simulink model "Decimator"  (R2023b)
settings: Solver=VariableStepAuto  StartTime=0.0  StopTime=10.0  RelTol=1e-3
PreLoadFcn:
  | startup
undefined symbols (not defined in the file): designMultirateFIR, fclk
libraries: hdlBasic x94, dspmlti4 x49, hdlsllib x2, simulink x2, dspbuff3 x2, dspsigops x2, hdlDSPIP x1, vmcUtilities x1
settings Model: Creator=andre  LastModifiedBy=andre

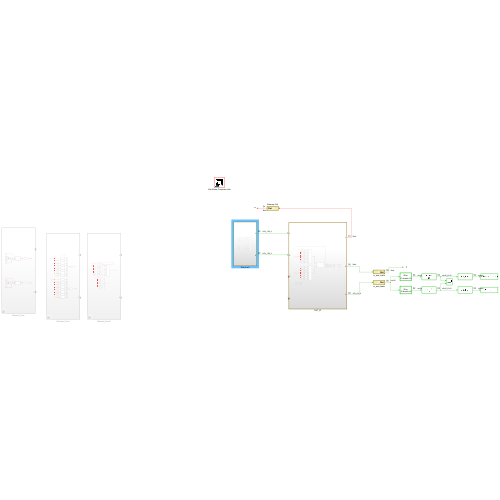
[thumbnail: Simulink's stored preview of the top-level diagram]
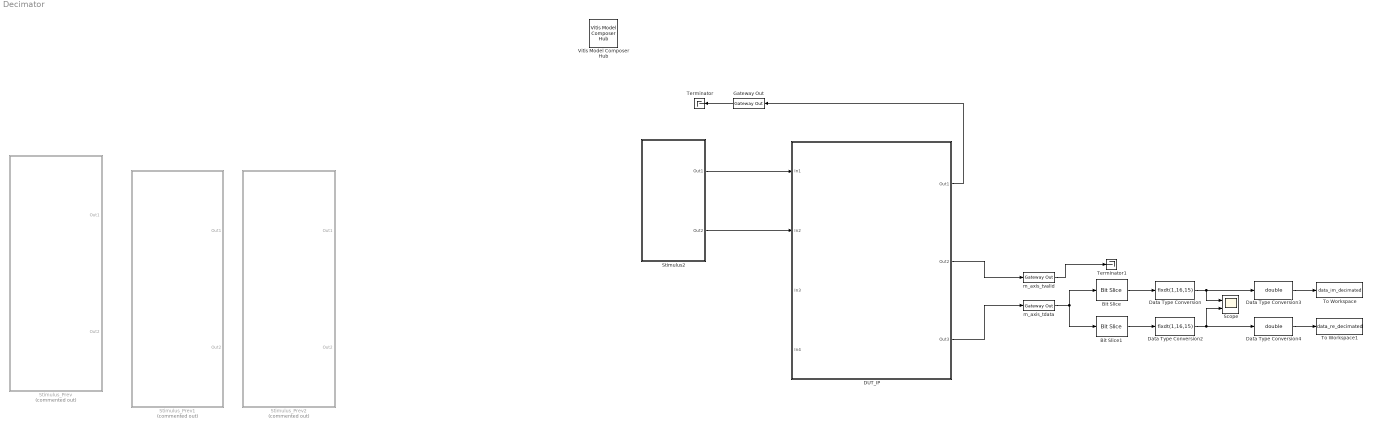
== system Decimator ==
  Bit Slice : hdlsllib/Logic and Bit Operations/Bit Slice  lidx=31  ridx=16
  Bit Slice1 : hdlsllib/Logic and Bit Operations/Bit Slice  lidx=15  ridx=0
  DUT_IP : Subsystem
  Data Type Conversion : DataTypeConversion  OutDataTypeStr=fixdt(1,16,15)  ConvertRealWorld=Stored Integer (SI)  SaturateOnIntegerOverflow=off  RndMeth=Floor
  Data Type Conversion2 : DataTypeConversion  OutDataTypeStr=fixdt(1,16,15)  ConvertRealWorld=Stored Integer (SI)  SaturateOnIntegerOverflow=off  RndMeth=Floor
  Data Type Conversion3 : DataTypeConversion  OutDataTypeStr=double  RndMeth=Floor
  Data Type Conversion4 : DataTypeConversion  OutDataTypeStr=double  RndMeth=Floor
  Gateway Out : hdlBasic/Gateway Out  inherit_from_input=off  hdl_port=on  rows=1  columns=1  UseAsDAC=off  DACChannel='1'  interface=None  automatic_assignment=on  address_offset=hex2dec('00')  intf_name=''  intf_description=''  timing_constraint=None  locs_specified=off  LOCs={}  io_standard={}  XmcBlockStatus=1  maskContainerNames=group4  block_type=gatewayout  block_config=sysgen:gateway_out_config  block_width_w=590  block_height_w=620  block_width=620  block_height=750
  Scope : Scope  NumInputPorts=2
  Stimulus2 : Subsystem
  Stimulus_Prev : Subsystem  Commented=on
  Stimulus_Prev1 : Subsystem  Commented=on
  Stimulus_Prev2 : Subsystem  Commented=on
  Terminator : Terminator
  Terminator1 : Terminator
  To Workspace : ToWorkspace  VariableName=data_im_decimated  SaveFormat=Timeseries  SampleTime=-1
  To Workspace1 : ToWorkspace  VariableName=data_re_decimated  SaveFormat=Timeseries  SampleTime=-1
  Vitis Model Composer Hub : vmcUtilities/Vitis Model Composer Hub  Tag=genX  CodeGeneration=off  SubsystemName=DUT_IP  DUTSubsystemName=DUT_IP  CompilationType=HDLCompilation  ExportTypeV2=IP Catalog  TargetDirectory=./netlist\ip\DUT_IP\src  exportDesign=on  analyzeDesign=off  validateDesignOnHw=off  ExportType=HDL  IpVendor=xilinx.com  IpLibrary=hls  IpVersion=1.0  IpHWLanguage=Verilog  AieCompilerOptions={}  AieSimulatorOptions={}  CreateTestbench=off  TestbenchStackSize=10  RunRtlSim=off  RunCSim=off  RunAieSim=off  AieSimTimeout=50000  RunAieSimProfiling=off  LaunchVitisAnalyzer=off  PlotOutput=off  RunX86Sim=off  X86SimTimeout=10  GenHwImage=off  GenLibadfXo=on  GenHwValidationCode=off  PlatformType=Not Specified  HwSystemType=Baremetal  HwValidationTarget=hw  ProjDevice=xczu28dr-ffvg1517-2-e  ProjDevicePart=xczu28dr-ffvg1517-2-e  SamplePeriod=-1  ClockFrequency=200  DataPathParallelism=1  xilinxfamily=zynquplusRFSOC  part=xczu28dr  speed=-2-e  package=ffvg1517  directory=./netlist\ip\DUT_IP\src  testbench=off  incr_netlist=off  synthesis_tool=Vivado  clock_wrapper=Clock Enables  dbl_ovrd=According to Block Masks  dcm_input_clock_period=10  sysclk_period=(1/fclk*8)*(1e6)  simulink_period=1/(fclk*8)  eval_field=0  IPInfoJsonString="{\"HDLSubsystem\":{\"SubsystemName\":\"DUT_IP\",\"IPName\":\"DUT_IP\",\"IPLibrary\":\"VMC\",\"IPVendor\":\"User Company\",\"IPVersion\":\"1.0\",\"TargetDirectory\":\"./netlist\",\"SubsystemDir\":\"./netlist\\\\ip\\\\DUT_IP\"},\"SubsystemTag\":\"HDLNode\"}"  LogFileName=''  NThreads=4
  m_axis_tdata : hdlBasic/Gateway Out  inherit_from_input=on  hdl_port=on  rows=1  columns=1  UseAsDAC=off  DACChannel='1'  interface=None  automatic_assignment=on  address_offset=hex2dec('00')  intf_name=''  intf_description=''  timing_constraint=None  locs_specified=off  LOCs={}  io_standard={}  XmcBlockStatus=1  maskContainerNames=group4  block_type=gatewayout  block_config=sysgen:gateway_out_config  block_width_w=590  block_height_w=620  block_width=620  block_height=750
  m_axis_tvalid : hdlBasic/Gateway Out  inherit_from_input=off  hdl_port=on  rows=1  columns=1  UseAsDAC=off  DACChannel='1'  interface=None  automatic_assignment=on  address_offset=hex2dec('00')  intf_name=''  intf_description=''  timing_constraint=None  locs_specified=off  LOCs={}  io_standard={}  XmcBlockStatus=1  maskContainerNames=group4  block_type=gatewayout  block_config=sysgen:gateway_out_config  block_width_w=590  block_height_w=620  block_width=620  block_height=750
  wires:
  Gateway Out/1 -> Terminator/1
  m_axis_tvalid/1 -> Terminator1/1
  m_axis_tdata/1 -> Bit Slice/1, Bit Slice1/1
  Bit Slice/1 -> Data Type Conversion/1
  Bit Slice1/1 -> Data Type Conversion2/1
  Data Type Conversion/1 -> Scope/1, Data Type Conversion3/1
  Data Type Conversion2/1 -> Scope/2, Data Type Conversion4/1
  Data Type Conversion3/1 -> To Workspace/1
  Data Type Conversion4/1 -> To Workspace1/1
  DUT_IP/1(Out1) -> Gateway Out/1
  DUT_IP/2(Out2) -> m_axis_tvalid/1
  DUT_IP/3(Out3) -> m_axis_tdata/1
  Stimulus2/1(Out1) -> DUT_IP/1(In1)
  Stimulus2/2(Out2) -> DUT_IP/2(In2)

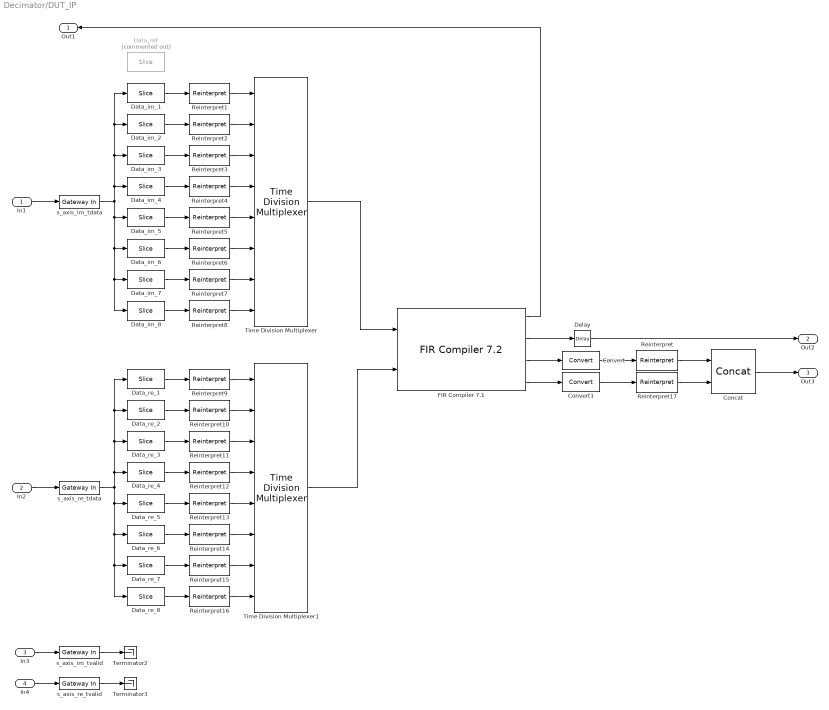
== system Decimator/DUT_IP ==
  In1 : Inport
  In2 : Inport  Port=2
  In3 : Inport  Port=3
  In4 : Inport  Port=4
  Concat : hdlBasic/Concat  num_inputs=2  XmcBlockStatus=1  maskContainerNames=group1  block_type=concat  block_config=sysgen:Concat_config
  Convert : hdlBasic/Convert  gui_display_data_type=Fixed-point  arith_type=Signed (2's comp)  n_bits=16  bin_pt=15  float_type=Single  exp_bits=8  fraction_bits=24  quantization=Truncate  overflow=Saturate  en=off  latency=1  pipeline=off  XmcBlockStatus=1  maskContainerNames=group2  block_type=convert  block_config=sysgen:Convert_config  block_width=595  block_height=885
  Convert1 : hdlBasic/Convert  gui_display_data_type=Fixed-point  arith_type=Signed (2's comp)  n_bits=16  bin_pt=15  float_type=Single  exp_bits=8  fraction_bits=24  quantization=Truncate  overflow=Saturate  en=off  latency=1  pipeline=off  XmcBlockStatus=1  maskContainerNames=group2  block_type=convert  block_config=sysgen:Convert_config  block_width=595  block_height=885
  Data_im_1 : hdlBasic/Slice  nbits=16  boolean_output=off  mode=Upper Bit Location + Width  bit1=127  base1=LSB of Input  bit0=16*8-(16*1)  base0=LSB of Input  XmcBlockStatus=1  maskContainerNames=group1  block_type=slice  block_config=sysgen:Slice_config
  Data_im_2 : hdlBasic/Slice  nbits=16  boolean_output=off  mode=Upper Bit Location + Width  bit1=111  base1=LSB of Input  bit0=16*8-(16*1)  base0=LSB of Input  XmcBlockStatus=1  maskContainerNames=group1  block_type=slice  block_config=sysgen:Slice_config
  Data_im_3 : hdlBasic/Slice  nbits=16  boolean_output=off  mode=Upper Bit Location + Width  bit1=95  base1=LSB of Input  bit0=16*8-(16*1)  base0=LSB of Input  XmcBlockStatus=1  maskContainerNames=group1  block_type=slice  block_config=sysgen:Slice_config
  Data_im_4 : hdlBasic/Slice  nbits=16  boolean_output=off  mode=Upper Bit Location + Width  bit1=79  base1=LSB of Input  bit0=16*8-(16*1)  base0=LSB of Input  XmcBlockStatus=1  maskContainerNames=group1  block_type=slice  block_config=sysgen:Slice_config
  Data_im_5 : hdlBasic/Slice  nbits=16  boolean_output=off  mode=Upper Bit Location + Width  bit1=63  base1=LSB of Input  bit0=16*8-(16*1)  base0=LSB of Input  XmcBlockStatus=1  maskContainerNames=group1  block_type=slice  block_config=sysgen:Slice_config
  Data_im_6 : hdlBasic/Slice  nbits=16  boolean_output=off  mode=Upper Bit Location + Width  bit1=47  base1=LSB of Input  bit0=16*8-(16*1)  base0=LSB of Input  XmcBlockStatus=1  maskContainerNames=group1  block_type=slice  block_config=sysgen:Slice_config
  Data_im_7 : hdlBasic/Slice  nbits=16  boolean_output=off  mode=Upper Bit Location + Width  bit1=31  base1=LSB of Input  bit0=16*8-(16*1)  base0=LSB of Input  XmcBlockStatus=1  maskContainerNames=group1  block_type=slice  block_config=sysgen:Slice_config
  Data_im_8 : hdlBasic/Slice  nbits=16  boolean_output=off  mode=Upper Bit Location + Width  bit1=15  base1=LSB of Input  bit0=16*8-(16*1)  base0=LSB of Input  XmcBlockStatus=1  maskContainerNames=group1  block_type=slice  block_config=sysgen:Slice_config
  Data_re_1 : hdlBasic/Slice  nbits=16  boolean_output=off  mode=Upper Bit Location + Width  bit1=127  base1=LSB of Input  bit0=16*8-(16*1)  base0=LSB of Input  XmcBlockStatus=1  maskContainerNames=group1  block_type=slice  block_config=sysgen:Slice_config
  Data_re_2 : hdlBasic/Slice  nbits=16  boolean_output=off  mode=Upper Bit Location + Width  bit1=111  base1=LSB of Input  bit0=16*8-(16*1)  base0=LSB of Input  XmcBlockStatus=1  maskContainerNames=group1  block_type=slice  block_config=sysgen:Slice_config
  Data_re_3 : hdlBasic/Slice  nbits=16  boolean_output=off  mode=Upper Bit Location + Width  bit1=95  base1=LSB of Input  bit0=16*8-(16*1)  base0=LSB of Input  XmcBlockStatus=1  maskContainerNames=group1  block_type=slice  block_config=sysgen:Slice_config
  Data_re_4 : hdlBasic/Slice  nbits=16  boolean_output=off  mode=Upper Bit Location + Width  bit1=79  base1=LSB of Input  bit0=16*8-(16*1)  base0=LSB of Input  XmcBlockStatus=1  maskContainerNames=group1  block_type=slice  block_config=sysgen:Slice_config
  Data_re_5 : hdlBasic/Slice  nbits=16  boolean_output=off  mode=Upper Bit Location + Width  bit1=63  base1=LSB of Input  bit0=16*8-(16*1)  base0=LSB of Input  XmcBlockStatus=1  maskContainerNames=group1  block_type=slice  block_config=sysgen:Slice_config
  Data_re_6 : hdlBasic/Slice  nbits=16  boolean_output=off  mode=Upper Bit Location + Width  bit1=47  base1=LSB of Input  bit0=16*8-(16*1)  base0=LSB of Input  XmcBlockStatus=1  maskContainerNames=group1  block_type=slice  block_config=sysgen:Slice_config
  Data_re_7 : hdlBasic/Slice  nbits=16  boolean_output=off  mode=Upper Bit Location + Width  bit1=31  base1=LSB of Input  bit0=16*8-(16*1)  base0=LSB of Input  XmcBlockStatus=1  maskContainerNames=group1  block_type=slice  block_config=sysgen:Slice_config
  Data_re_8 : hdlBasic/Slice  nbits=16  boolean_output=off  mode=Upper Bit Location + Width  bit1=15  base1=LSB of Input  bit0=16*8-(16*1)  base0=LSB of Input  XmcBlockStatus=1  maskContainerNames=group1  block_type=slice  block_config=sysgen:Slice_config
  Data_ref : hdlBasic/Slice  Commented=on  nbits=16  boolean_output=off  mode=Two Bit Locations  bit1=127  base1=LSB of Input  bit0=112  base0=LSB of Input  XmcBlockStatus=1  maskContainerNames=group1  block_type=slice  block_config=sysgen:Slice_config
  Delay : hdlBasic/Delay  rst=off  en=off  latency=1  reg_retiming=off  XmcBlockStatus=1  maskContainerNames=group1  block_type=delay  block_config=sysgen:Delay_config
  FIR Compiler 7.1 : hdlDSPIP/FIR Compiler 7.2   coefficientvector=src.getFilters.Stage1.Numerator  coefficient_sets=1  coefficient_reload=off  filter_type=Decimation  rate_change_type=Integer  interpolation_rate=1  decimation_rate=8  zero_pack_factor=1  channel_sequence=Basic  number_channels=1  pattern_list='P4-0,P4-1,P4-2,P4-3,P4-4'  number_paths=2  ratespecification=Maximum_Possible  sampleperiod=1  hardwareoversamplingrate=1  coefficient_sign=Signed  quantization=Quantize_Only  coefficient_width=16  bestprecision=on  coefficient_fractional_bits=15  coefficient_structure=Inferred  output_rounding_mode=Full_Precision  output_width=32  filter_architecture=Systolic_Multiply_Accumulate  optimization_goal=Area  optimization_list='None'  data_buffer_type=Automatic  coefficient_buffer_type=Automatic  input_buffer_type=Automatic  output_buffer_type=Automatic  preference_for_other_storage=Automatic  multi_column_support=Automatic  columnconfig='1'  inter_column_pipe_length=4  data_has_tlast=Not_Required  m_data_has_tready=off  s_data_has_fifo=off  s_data_has_tuser=Not_Required  m_data_has_tuser=Not_Required  s_config_sync_mode=On_Vector  s_config_method=Single  num_reload_slots=1  has_aclken=off  has_aresetn=off  reset_data_vector=on  trim_axipin_name=on  simulation_type=hybrid_sim  simulation_model=sysgen:xfirv7_2_cmodel  data_path_portlist={ 's_axis_data_tdata', 'm_axis_data_tdata' }  passband_min=0.0  passband_max=0.5  stopband_min=0.5  stopband_max=1.0  filter_selection=1  gui_behaviour='Sysgen_GUI'  data_sign=Signed  data_width=16  data_fractional_bits=0  data_tuser_width=1  wrapper_available=true  ip_wrap_arbitrary_binary_point=true  ip_name=FIR Compiler  ip_version=7.2  dsptool_ready=true  ipcore_usecache=true  ipcore_useipmodelcache=true  port_translation_map={ 'aclken' => 'en', 'aresetn' => 'rst' }  run_core_at_system_period=true  ipcore_xco_need_fpga_part=true  ipcore_fpga_part=[]  XmcBlockStatus=1  maskContainerNames=tabcontainer1  block_type=fir_compiler_v7_2  block_config=sysgen:rodinimport_config  block_width=820  block_height=600
  Reinterpret : hdlBasic/Reinterpret  force_arith_type=on  arith_type=Unsigned  force_bin_pt=on  bin_pt=0  XmcBlockStatus=1  maskContainerNames=group1  block_type=reinterpret  block_config=sysgen:Reinterpret_config
  Reinterpret{1..16} (16 alike) : hdlBasic/Reinterpret  force_arith_type=on  arith_type="Signed  (2's comp)"  force_bin_pt=on  bin_pt=15  XmcBlockStatus=1  maskContainerNames=group1  block_type=reinterpret  block_config=sysgen:Reinterpret_config
  Reinterpret17 : hdlBasic/Reinterpret  force_arith_type=on  arith_type=Unsigned  force_bin_pt=on  bin_pt=0  XmcBlockStatus=1  maskContainerNames=group1  block_type=reinterpret  block_config=sysgen:Reinterpret_config
  Terminator2 : Terminator
  Terminator3 : Terminator
  Time Division Multiplexer : hdlBasic/Time Division Multiplexer  inputs=8  vin=off  Optimization=Resource  explicit_period=off  period=1  XmcBlockStatus=1  maskContainerNames=group3  block_type=tdm  block_config=sysgen:TDM_config
  Time Division Multiplexer1 : hdlBasic/Time Division Multiplexer  inputs=8  vin=off  Optimization=Resource  explicit_period=off  period=1  XmcBlockStatus=1  maskContainerNames=group3  block_type=tdm  block_config=sysgen:TDM_config
  s_axis_im_tdata : hdlBasic/Gateway In  gui_display_data_type=Fixed-point  arith_type=Signed (2's comp)  n_bits=16*8  bin_pt=0  preci_type=Single  exp_width=8  frac_width=24  rows=1  columns=1  quantization=Truncate  overflow=Saturate  period=1/fclk  UseAsADC=off  ADCChannel='1'  interface=None  automatic_assignment=on  address_offset=hex2dec('00')  intf_name=''  intf_description=''  default_value=0  timing_constraint=None  locs_specified=off  LOCs={}  io_standard={}  inherit_from_input=off  hdl_port=on  XmcBlockStatus=1  maskContainerNames=group4  block_type=gatewayin  block_config=sysgen:gateway_in_config  block_width_w=590  block_height_w=620  block_width=640  block_height=850
  s_axis_im_tvalid : hdlBasic/Gateway In  gui_display_data_type=Boolean  arith_type=Boolean  n_bits=32  bin_pt=0  preci_type=Single  exp_width=8  frac_width=24  rows=1  columns=1  quantization="Round  (unbiased: +/- Inf)"  overflow=Saturate  period=1/fclk  UseAsADC=off  ADCChannel='1'  interface=None  automatic_assignment=on  address_offset=hex2dec('00')  intf_name=''  intf_description=''  default_value=0  timing_constraint=None  locs_specified=off  LOCs={}  io_standard={}  inherit_from_input=off  hdl_port=on  XmcBlockStatus=1  maskContainerNames=group4  block_type=gatewayin  block_config=sysgen:gateway_in_config  block_width_w=590  block_height_w=620  block_width=640  block_height=850
  s_axis_re_tdata : hdlBasic/Gateway In  gui_display_data_type=Fixed-point  arith_type=Signed (2's comp)  n_bits=16*8  bin_pt=0  preci_type=Single  exp_width=8  frac_width=24  rows=1  columns=1  quantization=Truncate  overflow=Saturate  period=1/fclk  UseAsADC=off  ADCChannel='1'  interface=None  automatic_assignment=on  address_offset=hex2dec('00')  intf_name=''  intf_description=''  default_value=0  timing_constraint=None  locs_specified=off  LOCs={}  io_standard={}  inherit_from_input=off  hdl_port=on  XmcBlockStatus=1  maskContainerNames=group4  block_type=gatewayin  block_config=sysgen:gateway_in_config  block_width_w=590  block_height_w=620  block_width=640  block_height=850
  s_axis_re_tvalid : hdlBasic/Gateway In  gui_display_data_type=Boolean  arith_type=Boolean  n_bits=32  bin_pt=0  preci_type=Single  exp_width=8  frac_width=24  rows=1  columns=1  quantization="Round  (unbiased: +/- Inf)"  overflow=Saturate  period=1/fclk  UseAsADC=off  ADCChannel='1'  interface=None  automatic_assignment=on  address_offset=hex2dec('00')  intf_name=''  intf_description=''  default_value=0  timing_constraint=None  locs_specified=off  LOCs={}  io_standard={}  inherit_from_input=off  hdl_port=on  XmcBlockStatus=1  maskContainerNames=group4  block_type=gatewayin  block_config=sysgen:gateway_in_config  block_width_w=590  block_height_w=620  block_width=640  block_height=850
  Out1 : Outport
  Out2 : Outport  Port=2
  Out3 : Outport  Port=3
  wires:
  Data_im_8/1 -> Reinterpret8/1
  Data_im_4/1 -> Reinterpret4/1
  In2/1 -> s_axis_re_tdata/1
  In1/1 -> s_axis_im_tdata/1
  Data_im_5/1 -> Reinterpret5/1
  Data_re_5/1 -> Reinterpret13/1
  FIR Compiler 7.1/2 -> Delay/1
  Reinterpret16/1 -> Time Division Multiplexer1/8
  Reinterpret13/1 -> Time Division Multiplexer1/5
  Reinterpret12/1 -> Time Division Multiplexer1/4
  Reinterpret14/1 -> Time Division Multiplexer1/6
  Data_re_7/1 -> Reinterpret15/1
  Data_im_7/1 -> Reinterpret7/1
  FIR Compiler 7.1/3 -> Convert/1
  Reinterpret10/1 -> Time Division Multiplexer1/2
  Reinterpret17/1 -> Concat/2
  Convert/1 -> Reinterpret/1
  Reinterpret1/1 -> Time Division Multiplexer/1
  Reinterpret11/1 -> Time Division Multiplexer1/3
  Reinterpret15/1 -> Time Division Multiplexer1/7
  FIR Compiler 7.1/1 -> Out1/1
  Reinterpret3/1 -> Time Division Multiplexer/3
  Reinterpret9/1 -> Time Division Multiplexer1/1
  Reinterpret4/1 -> Time Division Multiplexer/4
  Data_re_6/1 -> Reinterpret14/1
  Data_re_1/1 -> Reinterpret9/1
  Delay/1 -> Out2/1
  Time Division Multiplexer/1 -> FIR Compiler 7.1/1
  Data_re_8/1 -> Reinterpret16/1
  Data_re_4/1 -> Reinterpret12/1
  Convert1/1 -> Reinterpret17/1
  Data_re_2/1 -> Reinterpret10/1
  Concat/1 -> Out3/1
  Data_re_3/1 -> Reinterpret11/1
  Reinterpret7/1 -> Time Division Multiplexer/7
  Data_im_2/1 -> Reinterpret2/1
  Reinterpret2/1 -> Time Division Multiplexer/2
  Data_im_1/1 -> Reinterpret1/1
  Data_im_3/1 -> Reinterpret3/1
  Reinterpret8/1 -> Time Division Multiplexer/8
  Data_im_6/1 -> Reinterpret6/1
  Reinterpret5/1 -> Time Division Multiplexer/5
  Time Division Multiplexer1/1 -> FIR Compiler 7.1/2
  FIR Compiler 7.1/4 -> Convert1/1
  Reinterpret6/1 -> Time Division Multiplexer/6
  Reinterpret/1 -> Concat/1
  s_axis_im_tdata/1 -> Data_im_5/1, Data_im_6/1, Data_im_7/1, Data_im_8/1, Data_im_4/1, Data_im_3/1, Data_im_2/1, Data_im_1/1
  s_axis_re_tdata/1 -> Data_re_4/1, Data_re_3/1, Data_re_2/1, Data_re_1/1, Data_re_5/1, Data_re_6/1, Data_re_8/1, Data_re_7/1
  s_axis_re_tvalid/1 -> Terminator3/1
  s_axis_im_tvalid/1 -> Terminator2/1
  In3/1 -> s_axis_im_tvalid/1
  In4/1 -> s_axis_re_tvalid/1

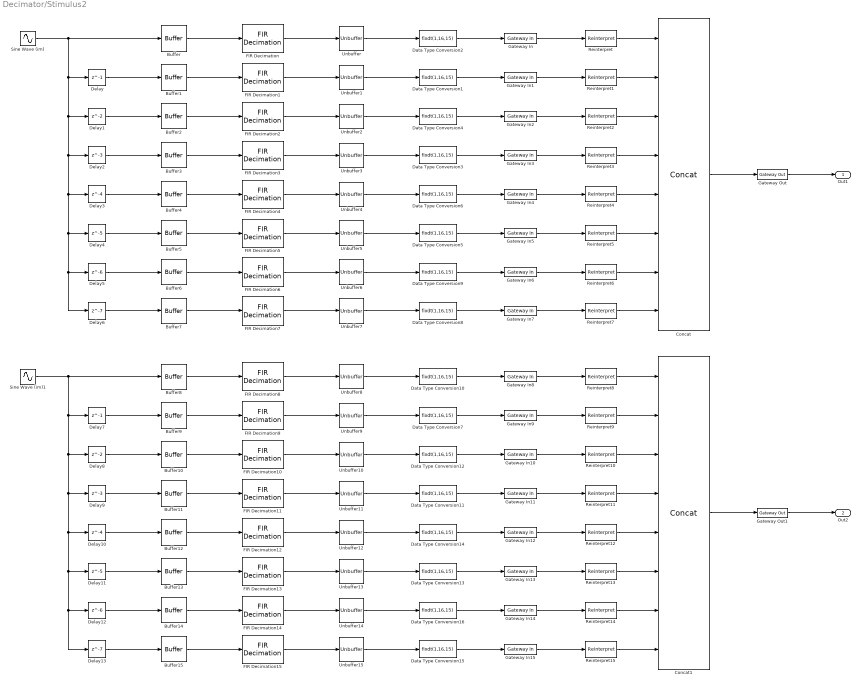
== system Decimator/Stimulus2 ==
  Buffer{,1..15} (16 alike) : Buffer  OutputFrames=off
  Concat : hdlBasic/Concat  num_inputs=8  XmcBlockStatus=1  maskContainerNames=group1  block_type=concat  block_config=sysgen:Concat_config
  Concat1 : hdlBasic/Concat  num_inputs=8  XmcBlockStatus=1  maskContainerNames=group1  block_type=concat  block_config=sysgen:Concat_config
  Data Type Conversion{1..16} (16 alike) : DataTypeConversion  OutDataTypeStr=fixdt(1,16,15)  RndMeth=Floor
  Delay : Delay  DelayLength=1  InitialCondition=0
  Delay1 : Delay  InitialCondition=0
  Delay10 : Delay  DelayLength=4  InitialCondition=0
  Delay11 : Delay  DelayLength=5  InitialCondition=0
  Delay12 : Delay  DelayLength=6  InitialCondition=0
  Delay13 : Delay  DelayLength=7  InitialCondition=0
  Delay2 : Delay  DelayLength=3  InitialCondition=0
  Delay3 : Delay  DelayLength=4  InitialCondition=0
  Delay4 : Delay  DelayLength=5  InitialCondition=0
  Delay5 : Delay  DelayLength=6  InitialCondition=0
  Delay6 : Delay  DelayLength=7  InitialCondition=0
  Delay7 : Delay  DelayLength=1  InitialCondition=0
  Delay8 : Delay  InitialCondition=0
  Delay9 : Delay  DelayLength=3  InitialCondition=0
  FIR Decimation{,1..15} (16 alike) : dspmlti4/FIR Decimation  FilterSource=Auto  h=designMultirateFIR(1,2)  D=8  filtStruct=Direct form  FilterObject=FDECIM  InputProcessing=Columns as channels (frame based)  framing=Enforce single-rate processing  AllowArbitraryInputLength=off  inputOffset=0  outputBufInitCond=0  roundingMode=Floor  overflowMode=off  firstCoeffDataTypeStr=Inherit: Same word length as input  firstCoeffMin=[]  firstCoeffMax=[]  firstCoeffLastDataTypeStr=Inherit: Same word length as input  outputDataTypeStr=Inherit: Same as accumulator  outputMin=[]  outputMax=[]  outputLastDataTypeStr=Inherit: Same as accumulator
  Gateway In{,1..15} (16 alike) : hdlBasic/Gateway In  gui_display_data_type=Fixed-point  arith_type=Signed (2's comp)  n_bits=16  bin_pt=15  preci_type=Single  exp_width=8  frac_width=24  rows=1  columns=1  quantization=Truncate  overflow=Saturate  period=1/(fclk)  UseAsADC=off  ADCChannel='1'  interface=None  automatic_assignment=on  address_offset=hex2dec('00')  intf_name=''  intf_description=''  default_value=0  timing_constraint=None  locs_specified=off  LOCs={}  io_standard={}  inherit_from_input=off  hdl_port=on  XmcBlockStatus=1  maskContainerNames=group4  block_type=gatewayin  block_config=sysgen:gateway_in_config  block_width_w=590  block_height_w=620  block_width=640  block_height=850
  Gateway Out : hdlBasic/Gateway Out  inherit_from_input=on  hdl_port=on  rows=1  columns=1  UseAsDAC=off  DACChannel='1'  interface=None  automatic_assignment=on  address_offset=hex2dec('00')  intf_name=''  intf_description=''  timing_constraint=None  locs_specified=off  LOCs={}  io_standard={}  XmcBlockStatus=1  maskContainerNames=group4  block_type=gatewayout  block_config=sysgen:gateway_out_config  block_width_w=590  block_height_w=620  block_width=620  block_height=750
  Gateway Out1 : hdlBasic/Gateway Out  inherit_from_input=on  hdl_port=on  rows=1  columns=1  UseAsDAC=off  DACChannel='1'  interface=None  automatic_assignment=on  address_offset=hex2dec('00')  intf_name=''  intf_description=''  timing_constraint=None  locs_specified=off  LOCs={}  io_standard={}  XmcBlockStatus=1  maskContainerNames=group4  block_type=gatewayout  block_config=sysgen:gateway_out_config  block_width_w=590  block_height_w=620  block_width=620  block_height=750
  Reinterpret{,1..15} (16 alike) : hdlBasic/Reinterpret  force_arith_type=on  arith_type=Unsigned  force_bin_pt=on  bin_pt=0  XmcBlockStatus=1  maskContainerNames=group1  block_type=reinterpret  block_config=sysgen:Reinterpret_config
  Sine Wave (im) : Sin  Amplitude=.2  Frequency=(3937e6)*pi  SampleTime=1/(fclk*8)
  Sine Wave (im)1 : Sin  Amplitude=.2  Frequency=(3937e6)*pi  SampleTime=1/(fclk*8)
  Unbuffer{,1..15} (16 alike) : Unbuffer
  Out1 : Outport
  Out2 : Outport  Port=2
  wires:
  Concat/1 -> Gateway Out/1
  Gateway Out/1 -> Out1/1
  Sine Wave (im)/1 -> Buffer/1, Delay6/1, Delay5/1, Delay4/1, Delay3/1, Delay2/1, Delay1/1, Delay/1
  Buffer/1 -> FIR Decimation/1
  Buffer1/1 -> FIR Decimation1/1
  Buffer2/1 -> FIR Decimation2/1
  Buffer3/1 -> FIR Decimation3/1
  Buffer7/1 -> FIR Decimation7/1
  Buffer6/1 -> FIR Decimation6/1
  Buffer5/1 -> FIR Decimation5/1
  Buffer4/1 -> FIR Decimation4/1
  Delay6/1 -> Buffer7/1
  Delay5/1 -> Buffer6/1
  Delay4/1 -> Buffer5/1
  Delay3/1 -> Buffer4/1
  Delay2/1 -> Buffer3/1
  Delay1/1 -> Buffer2/1
  Delay/1 -> Buffer1/1
  FIR Decimation/1 -> Unbuffer/1
  FIR Decimation1/1 -> Unbuffer1/1
  FIR Decimation3/1 -> Unbuffer3/1
  FIR Decimation2/1 -> Unbuffer2/1
  FIR Decimation6/1 -> Unbuffer6/1
  FIR Decimation7/1 -> Unbuffer7/1
  FIR Decimation5/1 -> Unbuffer5/1
  FIR Decimation4/1 -> Unbuffer4/1
  Unbuffer/1 -> Data Type Conversion2/1
  Unbuffer1/1 -> Data Type Conversion1/1
  Unbuffer3/1 -> Data Type Conversion3/1
  Unbuffer2/1 -> Data Type Conversion4/1
  Unbuffer6/1 -> Data Type Conversion9/1
  Unbuffer7/1 -> Data Type Conversion8/1
  Unbuffer5/1 -> Data Type Conversion5/1
  Unbuffer4/1 -> Data Type Conversion6/1
  Data Type Conversion2/1 -> Gateway In/1
  Data Type Conversion1/1 -> Gateway In1/1
  Data Type Conversion3/1 -> Gateway In3/1
  Data Type Conversion4/1 -> Gateway In2/1
  Data Type Conversion9/1 -> Gateway In6/1
  Data Type Conversion8/1 -> Gateway In7/1
  Data Type Conversion5/1 -> Gateway In5/1
  Data Type Conversion6/1 -> Gateway In4/1
  Gateway In/1 -> Reinterpret/1
  Gateway In1/1 -> Reinterpret1/1
  Gateway In3/1 -> Reinterpret3/1
  Gateway In2/1 -> Reinterpret2/1
  Gateway In6/1 -> Reinterpret6/1
  Gateway In7/1 -> Reinterpret7/1
  Gateway In5/1 -> Reinterpret5/1
  Gateway In4/1 -> Reinterpret4/1
  Reinterpret/1 -> Concat/1
  Reinterpret7/1 -> Concat/8
  Reinterpret1/1 -> Concat/2
  Reinterpret2/1 -> Concat/3
  Reinterpret3/1 -> Concat/4
  Reinterpret4/1 -> Concat/5
  Reinterpret5/1 -> Concat/6
  Reinterpret6/1 -> Concat/7
  Reinterpret14/1 -> Concat1/7
  Reinterpret13/1 -> Concat1/6
  Reinterpret12/1 -> Concat1/5
  Reinterpret11/1 -> Concat1/4
  Reinterpret10/1 -> Concat1/3
  Reinterpret9/1 -> Concat1/2
  Reinterpret15/1 -> Concat1/8
  Reinterpret8/1 -> Concat1/1
  Gateway In12/1 -> Reinterpret12/1
  Gateway In13/1 -> Reinterpret13/1
  Gateway In15/1 -> Reinterpret15/1
  Gateway In14/1 -> Reinterpret14/1
  Gateway In10/1 -> Reinterpret10/1
  Gateway In11/1 -> Reinterpret11/1
  Gateway In9/1 -> Reinterpret9/1
  Gateway In8/1 -> Reinterpret8/1
  Data Type Conversion14/1 -> Gateway In12/1
  Data Type Conversion13/1 -> Gateway In13/1
  Data Type Conversion15/1 -> Gateway In15/1
  Data Type Conversion16/1 -> Gateway In14/1
  Data Type Conversion12/1 -> Gateway In10/1
  Data Type Conversion11/1 -> Gateway In11/1
  Data Type Conversion7/1 -> Gateway In9/1
  Data Type Conversion10/1 -> Gateway In8/1
  Unbuffer12/1 -> Data Type Conversion14/1
  Unbuffer13/1 -> Data Type Conversion13/1
  Unbuffer15/1 -> Data Type Conversion15/1
  Unbuffer14/1 -> Data Type Conversion16/1
  Unbuffer10/1 -> Data Type Conversion12/1
  Unbuffer11/1 -> Data Type Conversion11/1
  Unbuffer9/1 -> Data Type Conversion7/1
  Unbuffer8/1 -> Data Type Conversion10/1
  FIR Decimation12/1 -> Unbuffer12/1
  FIR Decimation13/1 -> Unbuffer13/1
  FIR Decimation15/1 -> Unbuffer15/1
  FIR Decimation14/1 -> Unbuffer14/1
  FIR Decimation10/1 -> Unbuffer10/1
  FIR Decimation11/1 -> Unbuffer11/1
  FIR Decimation9/1 -> Unbuffer9/1
  FIR Decimation8/1 -> Unbuffer8/1
  Delay7/1 -> Buffer9/1
  Delay8/1 -> Buffer10/1
  Delay9/1 -> Buffer11/1
  Delay10/1 -> Buffer12/1
  Delay11/1 -> Buffer13/1
  Delay12/1 -> Buffer14/1
  Delay13/1 -> Buffer15/1
  Buffer12/1 -> FIR Decimation12/1
  Buffer13/1 -> FIR Decimation13/1
  Buffer14/1 -> FIR Decimation14/1
  Buffer15/1 -> FIR Decimation15/1
  Buffer11/1 -> FIR Decimation11/1
  Buffer10/1 -> FIR Decimation10/1
  Buffer9/1 -> FIR Decimation9/1
  Buffer8/1 -> FIR Decimation8/1
  Sine Wave (im)1/1 -> Delay7/1, Delay8/1, Delay9/1, Delay10/1, Delay11/1, Delay12/1, Delay13/1, Buffer8/1
  Gateway Out1/1 -> Out2/1
  Concat1/1 -> Gateway Out1/1

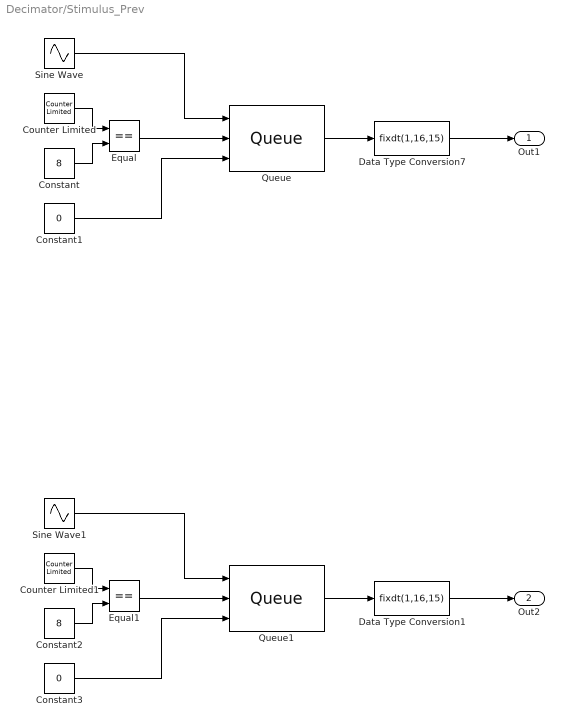
== system Decimator/Stimulus_Prev ==
  Constant : Constant  Value=8  SampleTime=1/fclk*8
  Constant1 : Constant  Value=0  OutDataTypeStr=boolean  SampleTime=1/fclk*8
  Constant2 : Constant  Value=8  SampleTime=1/fclk*8
  Constant3 : Constant  Value=0  SampleTime=1/fclk*8
  Counter Limited : simulink/Sources/Counter Limited  uplimit=8  tsamp=1/fclk*8
  Counter Limited1 : simulink/Sources/Counter Limited  uplimit=8  tsamp=1/fclk*8
  Data Type Conversion1 : DataTypeConversion  OutDataTypeStr=fixdt(1,16,15)  RndMeth=Floor
  Data Type Conversion7 : DataTypeConversion  OutDataTypeStr=fixdt(1,16,15)  RndMeth=Floor
  Equal : RelationalOperator  Operator===  OutDataTypeStr=boolean  RndMeth=Simplest  InputSameDT=off
  Equal1 : RelationalOperator  Operator===  OutDataTypeStr=boolean  RndMeth=Simplest  InputSameDT=off
  Queue : dspbuff3/Queue  depth=8  trigger=Rising edge  overflow=Dynamic reallocation  pes=Warning  eso=off  fso=off  nso=off  clr=off  clrOutport=off  adf=on
  Queue1 : dspbuff3/Queue  depth=8  trigger=Rising edge  overflow=Dynamic reallocation  pes=Warning  eso=off  fso=off  nso=off  clr=off  clrOutport=off  adf=on
  Sine Wave : Sin  Amplitude=.1  Frequency=(2e6)*2*pi  SampleTime=1/fclk*8
  Sine Wave1 : Sin  Amplitude=.1  Frequency=(2e6)*2*pi  Phase=pi/2  SampleTime=1/fclk*8
  Out1 : Outport
  Out2 : Outport  Port=2
  wires:
  Sine Wave/1 -> Queue/1
  Queue1/1 -> Data Type Conversion1/1
  Sine Wave1/1 -> Queue1/1
  Queue/1 -> Data Type Conversion7/1
  Constant2/1 -> Equal1/2
  Counter Limited1/1 -> Equal1/1
  Data Type Conversion7/1 -> Out1/1
  Constant1/1 -> Queue/3
  Equal1/1 -> Queue1/2
  Constant/1 -> Equal/2
  Counter Limited/1 -> Equal/1
  Equal/1 -> Queue/2
  Constant3/1 -> Queue1/3
  Data Type Conversion1/1 -> Out2/1

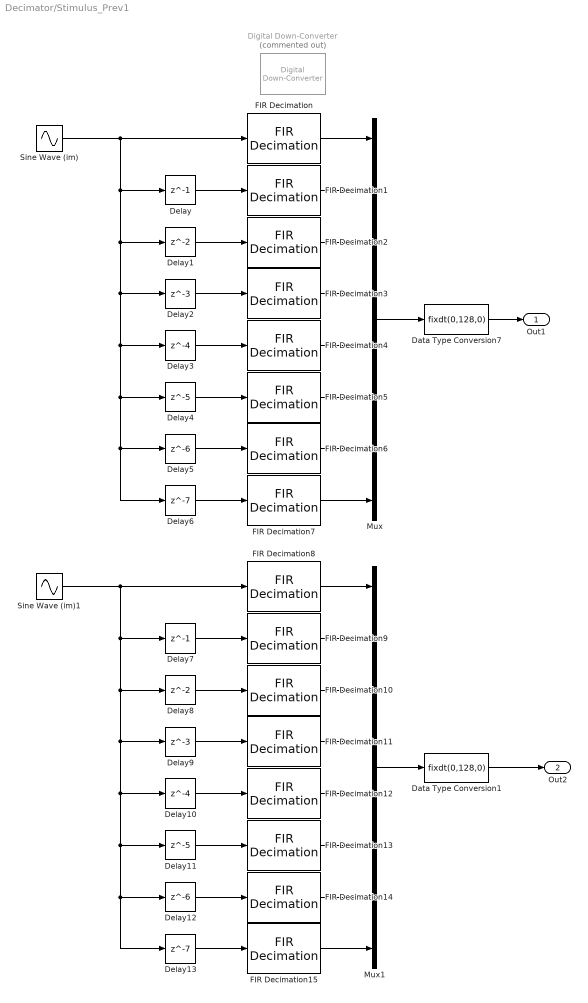
== system Decimator/Stimulus_Prev1 ==
  Data Type Conversion1 : DataTypeConversion  OutDataTypeStr=fixdt(0,128,0)  RndMeth=Floor
  Data Type Conversion7 : DataTypeConversion  OutDataTypeStr=fixdt(0,128,0)  RndMeth=Floor
  Delay : Delay  DelayLength=1  InitialCondition=0
  Delay1 : Delay  InitialCondition=0
  Delay10 : Delay  DelayLength=4  InitialCondition=0
  Delay11 : Delay  DelayLength=5  InitialCondition=0
  Delay12 : Delay  DelayLength=6  InitialCondition=0
  Delay13 : Delay  DelayLength=7  InitialCondition=0
  Delay2 : Delay  DelayLength=3  InitialCondition=0
  Delay3 : Delay  DelayLength=4  InitialCondition=0
  Delay4 : Delay  DelayLength=5  InitialCondition=0
  Delay5 : Delay  DelayLength=6  InitialCondition=0
  Delay6 : Delay  DelayLength=7  InitialCondition=0
  Delay7 : Delay  DelayLength=1  InitialCondition=0
  Delay8 : Delay  InitialCondition=0
  Delay9 : Delay  DelayLength=3  InitialCondition=0
  Digital Down-Converter : dspsigops/Digital Down-Converter  Commented=on  DecimationFactor=100  MinimumOrderDesign=on  NumCICSections=3  ThirdFilterOrder=10  StopbandFrequencySource=Auto  Oscillator=Sine wave  CenterFrequency=14e6  SecondFilterOrder=12  Bandwidth=200000  StopbandFrequency=150000  PassbandRipple=0.1  StopbandAttenuation=60  NumAccumulatorBits=16  NumQuantizedAccumulatorBits=12  Dither=on  NumDitherBits=4  InheritSampleRate=off  SampleRate=1/fclk*8  SimulateUsing=Code generation  outputMin=[]  outputMax=[]
  FIR Decimation{,1..15} (16 alike) : dspmlti4/FIR Decimation  FilterSource=Auto  h=designMultirateFIR(1,2)  D=8  filtStruct=Direct form  FilterObject=FDECIM  framing=Enforce single-rate processing  AllowArbitraryInputLength=off  inputOffset=0  outputBufInitCond=0  roundingMode=Floor  overflowMode=off  firstCoeffDataTypeStr=Inherit: Same word length as input  firstCoeffMin=[]  firstCoeffMax=[]  firstCoeffLastDataTypeStr=Inherit: Same word length as input  outputDataTypeStr=Inherit: Same as accumulator  outputMin=[]  outputMax=[]  outputLastDataTypeStr=Inherit: Same as accumulator
  Mux : Mux  Inputs=8
  Mux1 : Mux  Inputs=8
  Sine Wave (im) : Sin  Amplitude=.1  Frequency=(2e6)*2*pi  SampleTime=1/fclk*8
  Sine Wave (im)1 : Sin  Amplitude=.1  Frequency=(2e6)*2*pi  Phase=pi/2  SampleTime=1/fclk*8
  Out1 : Outport
  Out2 : Outport  Port=2
  wires:
  Data Type Conversion1/1 -> Out2/1
  Data Type Conversion7/1 -> Out1/1
  Sine Wave (im)/1 -> FIR Decimation/1, Delay6/1, Delay5/1, Delay4/1, Delay3/1, Delay2/1, Delay1/1, Delay/1
  FIR Decimation1/1 -> Mux/2
  FIR Decimation2/1 -> Mux/3
  FIR Decimation3/1 -> Mux/4
  FIR Decimation4/1 -> Mux/5
  FIR Decimation5/1 -> Mux/6
  FIR Decimation7/1 -> Mux/8
  Mux/1 -> Data Type Conversion7/1
  FIR Decimation6/1 -> Mux/7
  Delay/1 -> FIR Decimation1/1
  Delay1/1 -> FIR Decimation2/1
  Delay2/1 -> FIR Decimation3/1
  Delay3/1 -> FIR Decimation4/1
  Delay4/1 -> FIR Decimation5/1
  Delay5/1 -> FIR Decimation6/1
  Delay6/1 -> FIR Decimation7/1
  Delay13/1 -> FIR Decimation15/1
  Delay12/1 -> FIR Decimation14/1
  Delay11/1 -> FIR Decimation13/1
  Delay10/1 -> FIR Decimation12/1
  Delay9/1 -> FIR Decimation11/1
  Delay8/1 -> FIR Decimation10/1
  Delay7/1 -> FIR Decimation9/1
  FIR Decimation14/1 -> Mux1/7
  Mux1/1 -> Data Type Conversion1/1
  FIR Decimation15/1 -> Mux1/8
  FIR Decimation13/1 -> Mux1/6
  FIR Decimation12/1 -> Mux1/5
  FIR Decimation11/1 -> Mux1/4
  FIR Decimation10/1 -> Mux1/3
  FIR Decimation9/1 -> Mux1/2
  FIR Decimation8/1 -> Mux1/1
  Sine Wave (im)1/1 -> Delay7/1, Delay8/1, Delay9/1, Delay10/1, Delay11/1, Delay12/1, Delay13/1, FIR Decimation8/1
  FIR Decimation/1 -> Mux/1

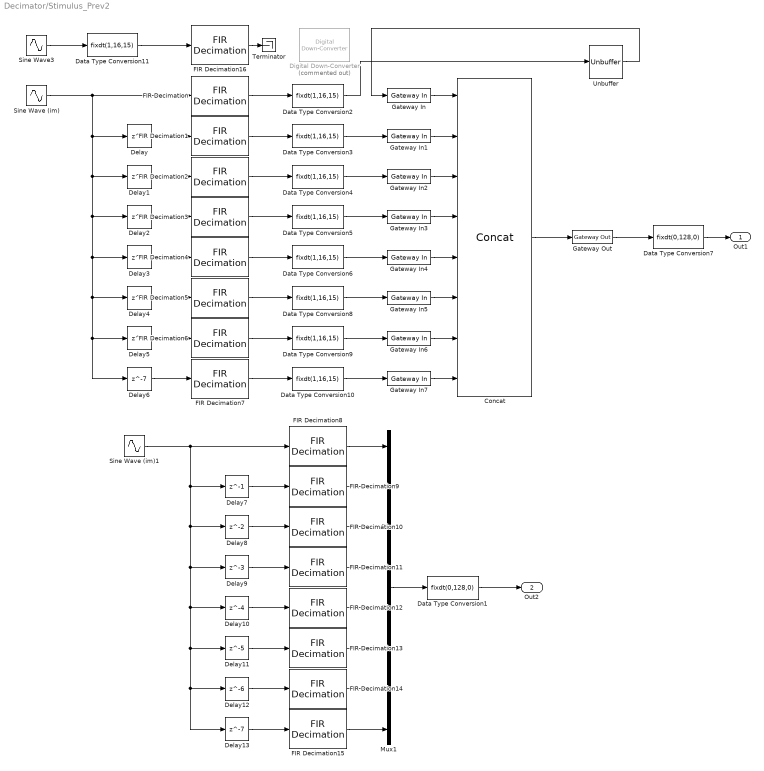
== system Decimator/Stimulus_Prev2 ==
  Concat : hdlBasic/Concat  num_inputs=8  XmcBlockStatus=1  maskContainerNames=group1  block_type=concat  block_config=sysgen:Concat_config
  Data Type Conversion1 : DataTypeConversion  OutDataTypeStr=fixdt(0,128,0)  RndMeth=Floor
  Data Type Conversion{2..6,8..11} (9 alike) : DataTypeConversion  OutDataTypeStr=fixdt(1,16,15)  RndMeth=Floor
  Data Type Conversion7 : DataTypeConversion  OutDataTypeStr=fixdt(0,128,0)  RndMeth=Floor
  Delay : Delay  DelayLength=1  InitialCondition=0
  Delay1 : Delay  InitialCondition=0
  Delay10 : Delay  DelayLength=4  InitialCondition=0
  Delay11 : Delay  DelayLength=5  InitialCondition=0
  Delay12 : Delay  DelayLength=6  InitialCondition=0
  Delay13 : Delay  DelayLength=7  InitialCondition=0
  Delay2 : Delay  DelayLength=3  InitialCondition=0
  Delay3 : Delay  DelayLength=4  InitialCondition=0
  Delay4 : Delay  DelayLength=5  InitialCondition=0
  Delay5 : Delay  DelayLength=6  InitialCondition=0
  Delay6 : Delay  DelayLength=7  InitialCondition=0
  Delay7 : Delay  DelayLength=1  InitialCondition=0
  Delay8 : Delay  InitialCondition=0
  Delay9 : Delay  DelayLength=3  InitialCondition=0
  Digital Down-Converter : dspsigops/Digital Down-Converter  Commented=on  DecimationFactor=100  MinimumOrderDesign=on  NumCICSections=3  ThirdFilterOrder=10  StopbandFrequencySource=Auto  Oscillator=Sine wave  CenterFrequency=14e6  SecondFilterOrder=12  Bandwidth=200000  StopbandFrequency=150000  PassbandRipple=0.1  StopbandAttenuation=60  NumAccumulatorBits=16  NumQuantizedAccumulatorBits=12  Dither=on  NumDitherBits=4  InheritSampleRate=off  SampleRate=1/fclk*8  SimulateUsing=Code generation  outputMin=[]  outputMax=[]
  FIR Decimation{,1..16} (17 alike) : dspmlti4/FIR Decimation  FilterSource=Auto  h=designMultirateFIR(1,2)  D=8  filtStruct=Direct form  FilterObject=FDECIM  framing=Enforce single-rate processing  AllowArbitraryInputLength=off  inputOffset=0  outputBufInitCond=0  roundingMode=Floor  overflowMode=off  firstCoeffDataTypeStr=Inherit: Same word length as input  firstCoeffMin=[]  firstCoeffMax=[]  firstCoeffLastDataTypeStr=Inherit: Same word length as input  outputDataTypeStr=Inherit: Same as accumulator  outputMin=[]  outputMax=[]  outputLastDataTypeStr=Inherit: Same as accumulator
  Gateway In{,1..7} (8 alike) : hdlBasic/Gateway In  gui_display_data_type=Fixed-point  arith_type=Signed (2's comp)  n_bits=16  bin_pt=15  preci_type=Single  exp_width=8  frac_width=24  rows=1  columns=1  quantization="Round  (unbiased: +/- Inf)"  overflow=Saturate  period=1/fclk  UseAsADC=off  ADCChannel='1'  interface=None  automatic_assignment=on  address_offset=hex2dec('00')  intf_name=''  intf_description=''  default_value=0  timing_constraint=None  locs_specified=off  LOCs={}  io_standard={}  inherit_from_input=off  hdl_port=on  XmcBlockStatus=1  maskContainerNames=group4  block_type=gatewayin  block_config=sysgen:gateway_in_config  block_width_w=590  block_height_w=620  block_width=640  block_height=850
  Gateway Out : hdlBasic/Gateway Out  inherit_from_input=off  hdl_port=on  rows=1  columns=1  UseAsDAC=off  DACChannel='1'  interface=None  automatic_assignment=on  address_offset=hex2dec('00')  intf_name=''  intf_description=''  timing_constraint=None  locs_specified=off  LOCs={}  io_standard={}  XmcBlockStatus=1  maskContainerNames=group4  block_type=gatewayout  block_config=sysgen:gateway_out_config  block_width_w=590  block_height_w=620  block_width=620  block_height=750
  Mux1 : Mux  Inputs=8
  Sine Wave (im) : Sin  Amplitude=.2  Frequency=(3937e6)*pi  SampleTime=1/(fclk*8)
  Sine Wave (im)1 : Sin  Amplitude=.1  Frequency=(3937e6)*pi  Phase=pi/2  SampleTime=1/fclk*8
  Sine Wave3 : Sin  Amplitude=.1  Frequency=(3937e6)*pi  SampleTime=1/fclk
  Terminator : Terminator
  Unbuffer : Unbuffer
  Out1 : Outport
  Out2 : Outport  Port=2
  wires:
  FIR Decimation/1 -> Data Type Conversion2/1
  Sine Wave (im)1/1 -> FIR Decimation8/1, Delay13/1, Delay12/1, Delay11/1, Delay10/1, Delay9/1, Delay8/1, Delay7/1
  FIR Decimation8/1 -> Mux1/1
  FIR Decimation9/1 -> Mux1/2
  FIR Decimation10/1 -> Mux1/3
  FIR Decimation11/1 -> Mux1/4
  FIR Decimation12/1 -> Mux1/5
  FIR Decimation13/1 -> Mux1/6
  FIR Decimation15/1 -> Mux1/8
  Mux1/1 -> Data Type Conversion1/1
  FIR Decimation14/1 -> Mux1/7
  Delay7/1 -> FIR Decimation9/1
  Delay8/1 -> FIR Decimation10/1
  Delay9/1 -> FIR Decimation11/1
  Delay10/1 -> FIR Decimation12/1
  Delay11/1 -> FIR Decimation13/1
  Delay12/1 -> FIR Decimation14/1
  Delay13/1 -> FIR Decimation15/1
  Delay6/1 -> FIR Decimation7/1
  Delay5/1 -> FIR Decimation6/1
  Delay4/1 -> FIR Decimation5/1
  Delay3/1 -> FIR Decimation4/1
  Delay2/1 -> FIR Decimation3/1
  Delay1/1 -> FIR Decimation2/1
  Delay/1 -> FIR Decimation1/1
  FIR Decimation6/1 -> Data Type Conversion9/1
  Gateway Out/1 -> Data Type Conversion7/1
  FIR Decimation7/1 -> Data Type Conversion10/1
  FIR Decimation5/1 -> Data Type Conversion8/1
  FIR Decimation4/1 -> Data Type Conversion6/1
  FIR Decimation3/1 -> Data Type Conversion5/1
  FIR Decimation2/1 -> Data Type Conversion4/1
  FIR Decimation1/1 -> Data Type Conversion3/1
  Sine Wave (im)/1 -> Delay/1, Delay1/1, Delay2/1, Delay3/1, Delay4/1, Delay5/1, Delay6/1, FIR Decimation/1
  Data Type Conversion7/1 -> Out1/1
  Data Type Conversion1/1 -> Out2/1
  Gateway In/1 -> Concat/1
  Gateway In1/1 -> Concat/2
  Gateway In2/1 -> Concat/3
  Gateway In3/1 -> Concat/4
  Gateway In4/1 -> Concat/5
  Gateway In5/1 -> Concat/6
  Gateway In6/1 -> Concat/7
  Gateway In7/1 -> Concat/8
  Concat/1 -> Gateway Out/1
  Unbuffer/1 -> Gateway In/1
  Data Type Conversion2/1 -> Unbuffer/1
  Data Type Conversion3/1 -> Gateway In1/1
  Data Type Conversion4/1 -> Gateway In2/1
  Data Type Conversion5/1 -> Gateway In3/1
  Data Type Conversion6/1 -> Gateway In4/1
  Data Type Conversion8/1 -> Gateway In5/1
  Data Type Conversion9/1 -> Gateway In6/1
  Data Type Conversion10/1 -> Gateway In7/1
  Sine Wave3/1 -> Data Type Conversion11/1
  Data Type Conversion11/1 -> FIR Decimation16/1
  FIR Decimation16/1 -> Terminator/1
